simulink model "gravity_model"  (R2021a)
settings: configuration reference "Configuration" (kept outside this file)
undefined symbols (not defined in the file): g, mq
settings Model: DataDictionary=shared_config.sldd  Creator=francois  LastModifiedBy=esl
settings ConfigSetRef: SourceName=Configuration

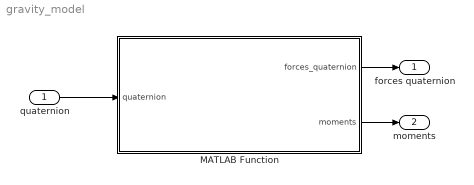
== system gravity_model ==
  quaternion : Inport  PortDimensions=4
  MATLAB Function : MATLAB Function  TreatAsAtomicUnit=on
  forces quaternion : Outport
  "moments " : Outport  Port=2
  wires:
  quaternion/1 -> MATLAB Function/1(quaternion)
  MATLAB Function/1(forces_quaternion) -> forces quaternion/1
  MATLAB Function/2(moments) -> "moments "/1

== matlab function gravity_model/MATLAB Function ==
  data: quaternion input; forces_quaternion output; moments output; mq parameter size=1; g parameter size=1
function [forces_quaternion, moments] = gravityModel(quaternion, mq, g)
    coder.extrinsic("quatrotate");
    
    % Initialize anders kla dit oor underspecified dimensions
    forces_quaternion = [0; 0; 0];

    forces_quaternion = quatrotate(quaternion', [0 ; 0 ; mq*g]')';
    
    moments = [0; 0; 0]; 
end
